simulink model "motorhomework_w2"  (R2023b)
settings: Solver=VariableStepAuto  StartTime=0.0  StopTime=0.1  RelTol=1e-3
values from neighbouring files (symbols this model uses):
  b = 0.1    [homeworkone.m]    (also in robotics_0911.m)
  J = 0.2    [homeworkone.m]    (also in robotics_0911.m)
  Ke = 1    [homeworkone.m]    (also in robotics_0911.m)
  Kt = 1    [homeworkone.m]    (also in robotics_0911.m)
  La = 1    [homeworkone.m]    (also in robotics_0911.m)
  Ra = 0.01    [homeworkone.m]    (also in robotics_0911.m)
  Va = 1    [homeworkone.m]    (also in robotics_0911.m)
undefined symbols (not defined in the file or in its folder): Tl_
settings Model: Creator=junseo  LastModifiedBy=minjs
settings OptimizationCC: ReuseModelBlockBuffer=off

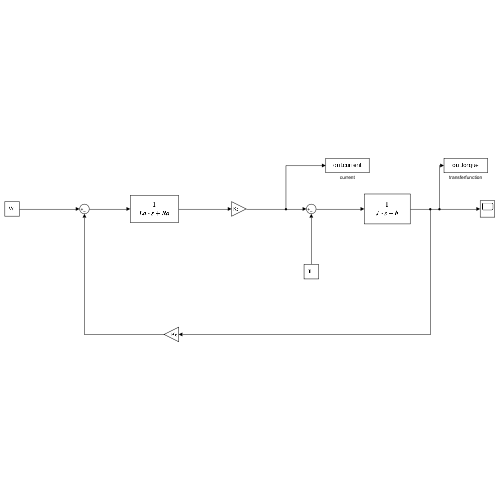
[thumbnail: Simulink's stored preview of the top-level diagram]
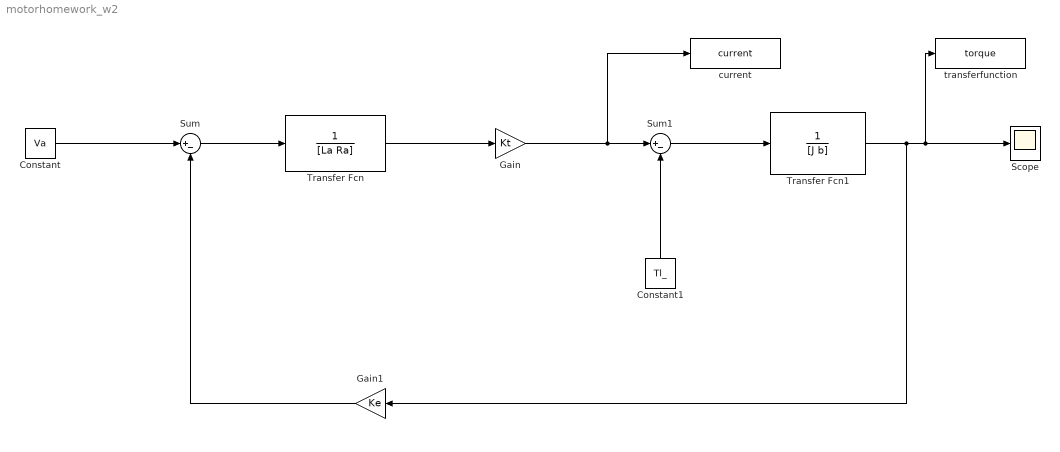
== system motorhomework_w2 ==
  Constant : Constant  Value=Va
  Constant1 : Constant  Value=Tl_
  Gain : Gain  Gain=Kt
  Gain1 : Gain  Gain=Ke
  Scope : Scope
  Sum : Sum  Inputs=|+-
  Sum1 : Sum  Inputs=|+-
  Transfer Fcn : TransferFcn  Denominator=[La Ra]
  Transfer Fcn1 : TransferFcn  Denominator=[J b]
  current : ToWorkspace  VariableName=current  SaveFormat=Timeseries  SampleTime=-1
  transferfunction : ToWorkspace  VariableName=torque  SaveFormat=Timeseries  SampleTime=-1
  wires:
  Constant/1 -> Sum/1
  Sum/1 -> Transfer Fcn/1
  Transfer Fcn/1 -> Gain/1
  Gain/1 -> Sum1/1, current/1
  Sum1/1 -> Transfer Fcn1/1
  Constant1/1 -> Sum1/2
  Transfer Fcn1/1 -> Gain1/1, transferfunction/1, Scope/1
  Gain1/1 -> Sum/2
